simulink model "Quad_F450_Model"  (R2023a)
settings: Solver=FixedStepAuto  StartTime=0.0  StopTime=inf  FixedStep=Copter.SimTs  RelTol=1e-3
InitFcn:
  | load("motor_data.mat")
  | run("Parameters.m")
undefined symbols (not defined in the file or in its folder): Controller, Copter, DiscIntNeverNeededParam, Earth, init, Keyboard, motor_data, w_der_filt, WGS84
libraries: sharedutil x12, slpidlib x8, sharedtransform x5, aerolibpropulsionsys x4, simulink_extras x3, matrix_library x3, shared6dof x1, aerolibtransform2 x1, aerolibatmos2 x1, aerolibsim3d x1, sim3dlib x1
(part 2 of 3)

== system Quad_F450_Model/Copter Properties/Arm_1 ==
  Bus Creator : BusCreator  Inputs=15
  Constant : Constant  Value=Copter.Arm1.Prop.R_m
  Constant1 : Constant  Value=Copter.Arm1.Prop.chord_m
  Constant10 : Constant  Value=Copter.Arm1.defect_rad
  Constant11 : Constant  Value=Copter.Arm1.Prop.Izz_kgm2
  Constant12 : Constant  Value=Copter.Arm1.Motor.time_constant_s
  Constant13 : Constant  Value=Copter.Arm1.Motor.pwm2rpm
  Constant14 : Constant  Value=Copter.Arm1.Prop.Direction
  Constant15 : Constant  Value=Copter.Arm1.h_cg2prop_m
  Constant2 : Constant  Value=Copter.Arm1.Prop.no_of_blades
  Constant3 : Constant  Value=Copter.Arm1.Prop.CT
  Constant4 : Constant  Value=Copter.Arm1.Prop.CQ
  Constant5 : Constant  Value=Copter.Arm1.Prop.flappingOffset_m
  Constant6 : Constant  Value=Copter.Arm1.Prop.Cl_alpha
  Constant7 : Constant  Value=Copter.Arm1.Prop.lock
  Constant8 : Constant  Value=Copter.Arm1.Prop.thetaTip_rad
  Constant9 : Constant  Value=Copter.Arm1.length_m
  Gain : Gain
  Gain1 : Gain
  Matrix Concatenate : Concatenate  NumInputs=3  ConcatenateDimension=2
  Arm_1 : Outport
  wires:
  Constant4/1 -> Bus Creator/10  "prop1_cq"
  Constant8/1 -> Bus Creator/14  "prop1_theta_tip_rad"
  Constant/1 -> Bus Creator/6  "prop1_radius_m"
  Constant2/1 -> Bus Creator/8  "prop1_no_of_blades"
  Constant3/1 -> Bus Creator/9  "prop1_ct"
  Constant6/1 -> Bus Creator/12  "prop1_Cl_alpha"
  Constant1/1 -> Bus Creator/7  "prop1_chord_m"
  Constant5/1 -> Bus Creator/11  "prop1_flapping_offset_m"
  Constant7/1 -> Bus Creator/13  "prop1_lock"
  Constant10/1 -> Bus Creator/2  "arm1_defect_rad"
  Constant11/1 -> Bus Creator/3  "prop1_Izz_kgm2"
  Constant12/1 -> Bus Creator/4  "motor1_time_constant_s"
  Constant13/1 -> Bus Creator/5  "motor1_pwm2rpm"
  Bus Creator/1 -> Arm_1/1
  Constant14/1 -> Bus Creator/15  "prop1_direction"
  Constant9/1 -> Gain1/1, Gain/1  "arm1_length_m"
  Constant15/1 -> Matrix Concatenate/3  "arm1_length_m"
  Gain/1 -> Matrix Concatenate/1
  Gain1/1 -> Matrix Concatenate/2
  Matrix Concatenate/1 -> Bus Creator/1  "cg2motor_arm1_m"

== system Quad_F450_Model/Copter Properties/Arm_2 ==
  Bus Creator : BusCreator  Inputs=15
  Constant : Constant  Value=Copter.Arm2.Prop.R_m
  Constant1 : Constant  Value=Copter.Arm2.Prop.chord_m
  Constant10 : Constant  Value=Copter.Arm2.defect_rad
  Constant11 : Constant  Value=Copter.Arm2.Prop.Izz_kgm2
  Constant12 : Constant  Value=Copter.Arm2.Motor.time_constant_s
  Constant13 : Constant  Value=Copter.Arm2.Motor.pwm2rpm
  Constant14 : Constant  Value=Copter.Arm2.Prop.Direction
  Constant15 : Constant  Value=Copter.Arm2.h_cg2prop_m
  Constant2 : Constant  Value=Copter.Arm2.Prop.no_of_blades
  Constant3 : Constant  Value=Copter.Arm2.Prop.CT
  Constant4 : Constant  Value=Copter.Arm2.Prop.CQ
  Constant5 : Constant  Value=Copter.Arm2.Prop.flappingOffset_m
  Constant6 : Constant  Value=Copter.Arm2.Prop.Cl_alpha
  Constant7 : Constant  Value=Copter.Arm2.Prop.lock
  Constant8 : Constant  Value=Copter.Arm2.Prop.thetaTip_rad
  Constant9 : Constant  Value=Copter.Arm2.length_m
  Gain : Gain  Gain=-1
  Gain1 : Gain  Gain=-1
  Matrix Concatenate : Concatenate  NumInputs=3  ConcatenateDimension=2
  Arm_2 : Outport
  wires:
  Constant4/1 -> Bus Creator/10  "prop2_cq"
  Constant8/1 -> Bus Creator/14  "prop2_theta_tip_rad"
  Constant/1 -> Bus Creator/6  "prop2_radius_m"
  Constant2/1 -> Bus Creator/8  "prop2_no_of_blades"
  Constant3/1 -> Bus Creator/9  "prop2_ct"
  Constant6/1 -> Bus Creator/12  "prop2_Cl_alpha"
  Constant1/1 -> Bus Creator/7  "prop2_chord_m"
  Constant5/1 -> Bus Creator/11  "prop2_flapping_offset_m"
  Constant7/1 -> Bus Creator/13  "prop2_lock"
  Constant10/1 -> Bus Creator/2  "arm2_defect_rad"
  Constant11/1 -> Bus Creator/3  "prop2_Izz_kgm2"
  Constant12/1 -> Bus Creator/4  "motor2_time_constant_s"
  Constant13/1 -> Bus Creator/5  "motor2_pwm2rpm"
  Bus Creator/1 -> Arm_2/1
  Constant14/1 -> Bus Creator/15  "prop2_direction"
  Constant9/1 -> Gain1/1, Gain/1  "arm2_length_m"
  Constant15/1 -> Matrix Concatenate/3  "arm2_length_m"
  Gain/1 -> Matrix Concatenate/1
  Gain1/1 -> Matrix Concatenate/2
  Matrix Concatenate/1 -> Bus Creator/1  "cg2motor_arm2_m"

== system Quad_F450_Model/Copter Properties/Arm_3 ==
  Bus Creator : BusCreator  Inputs=15
  Constant : Constant  Value=Copter.Arm3.Prop.R_m
  Constant1 : Constant  Value=Copter.Arm3.Prop.chord_m
  Constant10 : Constant  Value=Copter.Arm3.defect_rad
  Constant11 : Constant  Value=Copter.Arm3.Prop.Izz_kgm2
  Constant12 : Constant  Value=Copter.Arm3.Motor.time_constant_s
  Constant13 : Constant  Value=Copter.Arm3.Motor.pwm2rpm
  Constant14 : Constant  Value=Copter.Arm3.Prop.Direction
  Constant15 : Constant  Value=Copter.Arm3.h_cg2prop_m
  Constant2 : Constant  Value=Copter.Arm3.Prop.no_of_blades
  Constant3 : Constant  Value=Copter.Arm3.Prop.CT
  Constant4 : Constant  Value=Copter.Arm3.Prop.CQ
  Constant5 : Constant  Value=Copter.Arm3.Prop.flappingOffset_m
  Constant6 : Constant  Value=Copter.Arm3.Prop.Cl_alpha
  Constant7 : Constant  Value=Copter.Arm3.Prop.lock
  Constant8 : Constant  Value=Copter.Arm3.Prop.thetaTip_rad
  Constant9 : Constant  Value=Copter.Arm3.length_m
  Gain : Gain
  Gain1 : Gain  Gain=-1
  Matrix Concatenate : Concatenate  NumInputs=3  ConcatenateDimension=2
  Arm_3 : Outport
  wires:
  Constant4/1 -> Bus Creator/10  "prop3_cq"
  Constant8/1 -> Bus Creator/14  "prop3_theta_tip_rad"
  Constant/1 -> Bus Creator/6  "prop3_radius_m"
  Constant2/1 -> Bus Creator/8  "prop3_no_of_blades"
  Constant3/1 -> Bus Creator/9  "prop3_ct"
  Constant6/1 -> Bus Creator/12  "prop3_Cl_alpha"
  Constant1/1 -> Bus Creator/7  "prop3_chord_m"
  Constant5/1 -> Bus Creator/11  "prop3_flapping_offset_m"
  Constant7/1 -> Bus Creator/13  "prop3_lock"
  Constant10/1 -> Bus Creator/2  "arm3_defect_rad"
  Constant11/1 -> Bus Creator/3  "prop3_Izz_kgm2"
  Constant12/1 -> Bus Creator/4  "motor3_time_constant_s"
  Constant13/1 -> Bus Creator/5  "motor3_pwm2rpm"
  Bus Creator/1 -> Arm_3/1
  Constant14/1 -> Bus Creator/15  "prop3_direction"
  Constant9/1 -> Gain1/1, Gain/1  "arm3_length_m"
  Constant15/1 -> Matrix Concatenate/3  "arm3_length_m"
  Gain/1 -> Matrix Concatenate/1
  Gain1/1 -> Matrix Concatenate/2
  Matrix Concatenate/1 -> Bus Creator/1  "cg2motor_arm3_m"

== system Quad_F450_Model/Copter Properties/Arm_4 ==
  Bus Creator : BusCreator  Inputs=15
  Constant : Constant  Value=Copter.Arm4.Prop.R_m
  Constant1 : Constant  Value=Copter.Arm4.Prop.chord_m
  Constant10 : Constant  Value=Copter.Arm4.defect_rad
  Constant11 : Constant  Value=Copter.Arm4.Prop.Izz_kgm2
  Constant12 : Constant  Value=Copter.Arm4.Motor.time_constant_s
  Constant13 : Constant  Value=Copter.Arm4.Motor.pwm2rpm
  Constant14 : Constant  Value=Copter.Arm4.Prop.Direction
  Constant15 : Constant  Value=Copter.Arm4.h_cg2prop_m
  Constant2 : Constant  Value=Copter.Arm4.Prop.no_of_blades
  Constant3 : Constant  Value=Copter.Arm4.Prop.CT
  Constant4 : Constant  Value=Copter.Arm4.Prop.CQ
  Constant5 : Constant  Value=Copter.Arm4.Prop.flappingOffset_m
  Constant6 : Constant  Value=Copter.Arm4.Prop.Cl_alpha
  Constant7 : Constant  Value=Copter.Arm4.Prop.lock
  Constant8 : Constant  Value=Copter.Arm4.Prop.thetaTip_rad
  Constant9 : Constant  Value=Copter.Arm4.length_m
  Gain : Gain  Gain=-1
  Gain1 : Gain
  Matrix Concatenate : Concatenate  NumInputs=3  ConcatenateDimension=2
  Arm_4 : Outport
  wires:
  Constant4/1 -> Bus Creator/10  "prop4_cq"
  Constant8/1 -> Bus Creator/14  "prop4_theta_tip_rad"
  Constant/1 -> Bus Creator/6  "prop4_radius_m"
  Constant2/1 -> Bus Creator/8  "prop4_no_of_blades"
  Constant3/1 -> Bus Creator/9  "prop4_ct"
  Constant6/1 -> Bus Creator/12  "prop4_Cl_alpha"
  Constant1/1 -> Bus Creator/7  "prop4_chord_m"
  Constant5/1 -> Bus Creator/11  "prop4_flapping_offset_m"
  Constant7/1 -> Bus Creator/13  "prop4_lock"
  Constant10/1 -> Bus Creator/2  "arm4_defect_rad"
  Constant11/1 -> Bus Creator/3  "prop4_Izz_kgm2"
  Constant12/1 -> Bus Creator/4  "motor4_time_constant_s"
  Constant13/1 -> Bus Creator/5  "motor4_pwm2rpm"
  Bus Creator/1 -> Arm_4/1
  Constant14/1 -> Bus Creator/15  "prop4_direction"
  Constant9/1 -> Gain1/1, Gain/1  "arm4_length_m"
  Constant15/1 -> Matrix Concatenate/3  "arm4_length_m"
  Gain/1 -> Matrix Concatenate/1
  Gain1/1 -> Matrix Concatenate/2
  Matrix Concatenate/1 -> Bus Creator/1  "cg2motor_arm4_m"

== system Quad_F450_Model/Copter Properties/Subsystem ==
  Bus Creator : BusCreator  Inputs=7
  Constant1 : Constant  Value=Copter.inertia_matrix_kgm2
  Constant2 : Constant  Value=Copter.S_area_m2
  Constant3 : Constant  Value=Copter.Cd
  Constant4 : Constant  Value=Copter.Ryz_cg2ac_m
  Constant5 : Constant  Value=Copter.Rxz_cg2ac_m
  Constant6 : Constant  Value=Copter.Rxy_cg2ac_m
  Constant9 : Constant  Value=Copter.mass_kg
  Copter_Frame : Outport
  wires:
  Constant9/1 -> Bus Creator/1  "mass_kg"
  Constant1/1 -> Bus Creator/2  "inertia_matrix_kgm2"
  Constant2/1 -> Bus Creator/3  "S_area_m2"
  Constant3/1 -> Bus Creator/4  "Cd"
  Constant4/1 -> Bus Creator/5  "Ryz_cg2ac_m"
  Bus Creator/1 -> Copter_Frame/1
  Constant5/1 -> Bus Creator/6  "Rxz_cg2ac_m"
  Constant6/1 -> Bus Creator/7  "Rxy_cg2ac_m"

== system Quad_F450_Model/DYNAMIC_MODEL/Aerodynamic Forces and Moments ==
  V_air_ms : Inport
  Environment : Inport  Port=2
  Copter : Inport  Port=3
  Add : Sum  Inputs=3
  Bus Selector : BusSelector  OutputSignals=Frame.S_area_m2,Frame.Cd,Frame.Rxy_cg2ac_m,Frame.Rxz_cg2ac_m,Frame.Ryz_cg2ac_m
  Bus Selector1 : BusSelector  OutputSignals=Atmosphere_Prop.air_density_kgm3
  Constant : Constant  Value=0
  Constant1 : Constant  Value=0
  Constant2 : Constant  Value=0
  Cross Product : matrix_library/Cross Product
  Cross Product1 : matrix_library/Cross Product
  Cross Product2 : matrix_library/Cross Product
  Gain : Gain  Gain=-1
  Gain1 : Gain  Gain=1/2
  Mux : Mux  Inputs=3
  Mux1 : Mux  Inputs=3
  Mux2 : Mux  Inputs=3
  Product : Product  Inputs=5
  Selector : Selector  InputPortWidth=3  IndexOptions=Index vector (dialog)  Indices=1  OutputSizes=1
  Selector1 : Selector  InputPortWidth=3  IndexOptions=Index vector (dialog)  Indices=2  OutputSizes=1
  Selector2 : Selector  InputPortWidth=3  IndexOptions=Index vector (dialog)  Indices=3  OutputSizes=1
  Sign : Signum
  Square : Math  Operator=square
  F_aero_b_N : Outport
  M_aero_b_Nm : Outport  Port=2
  wires:
  Square/1 -> Gain1/1
  V_air_ms/1 -> Square/1, Sign/1
  [S_m2] -> Product/4
  [Cd] -> Product/5
  [rho_kgm3] -> Product/3
  Gain1/1 -> Product/2
  Copter/1 -> Bus Selector/1
  Bus Selector/3 -> [Rxy_cg2ac_m]  "<Rxy_cg2ac_m>"
  Bus Selector/2 -> [Cd]  "<Cd>"
  Bus Selector/1 -> [S_m2]  "<S_area_m2>"
  Environment/1 -> Bus Selector1/1
  Bus Selector1/1 -> [rho_kgm3]  "<air_density_kgm3>"
  Bus Selector/4 -> [Rxz_cg2ac_m]  "<Rxz_cg2ac_m>"
  Bus Selector/5 -> [Ryz_cg2ac_m]  "<Ryz_cg2ac_m>"
  Product/1 -> Gain/1
  [F_aero_b_N] -> F_aero_b_N/1
  [F_aero_b_N] -> Selector/1
  Selector/1 -> Mux/1
  Constant/1 -> Mux/3, Mux/2
  Mux/1 -> Cross Product/2
  [Ryz_cg2ac_m] -> Cross Product/1
  [Rxz_cg2ac_m] -> Cross Product1/1
  Mux1/1 -> Cross Product1/2
  [F_aero_b_N] -> Selector1/1
  [F_aero_b_N] -> Selector2/1
  Mux2/1 -> Cross Product2/2
  [Rxy_cg2ac_m] -> Cross Product2/1
  Selector2/1 -> Mux2/3
  Constant2/1 -> Mux2/1, Mux2/2
  Selector1/1 -> Mux1/2
  Constant1/1 -> Mux1/3, Mux1/1
  Cross Product1/1 -> Add/2
  Cross Product2/1 -> Add/3
  Cross Product/1 -> Add/1
  Add/1 -> M_aero_b_Nm/1
  Sign/1 -> Product/1
  Gain/1 -> [F_aero_b_N]

== system Quad_F450_Model/DYNAMIC_MODEL/Gravity Force  ==
  dcm_e2b : Inport
  Environment : Inport  Port=2
  Copter : Inport  Port=3
  Bus Selector : BusSelector  OutputSignals=Frame.mass_kg
  Bus Selector1 : BusSelector  OutputSignals=gravity_e_mss
  Matrix Multiply : Product  Multiplication=Matrix(*)
  Product : Product
  F_grav_b_N : Outport
  wires:
  dcm_e2b/1 -> Matrix Multiply/1
  Environment/1 -> Bus Selector1/1
  Matrix Multiply/1 -> Product/1
  Product/1 -> F_grav_b_N/1
  Copter/1 -> Bus Selector/1
  Bus Selector/1 -> Product/2  "<mass_kg>"
  Bus Selector1/1 -> Matrix Multiply/2  "<gravity_e_mss>"

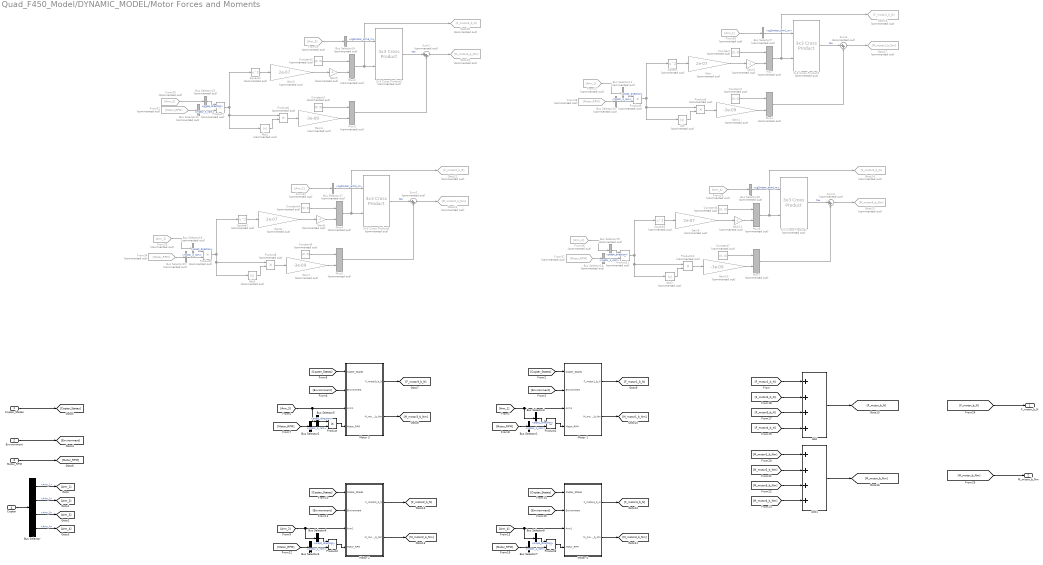
== system Quad_F450_Model/DYNAMIC_MODEL/Motor Forces and Moments ==
  Copter_States : Inport
  Environment : Inport  Port=2
  Motor_RPM : Inport  Port=3
  Copter : Inport  Port=4
  3x3 Cross Product{1..4} (4 alike) : sharedutil/3x3 Cross Product  Commented=on  aMode=aMode
      settings: LibrarySourceBlock=aerolibpropulsionsys/Rotor Subsystem/3x3 Cross Product1
  Abs{,1..3} (4 alike) : Abs  Commented=on  SaturateOnIntegerOverflow=off
  Add : Sum  Inputs=4
  Add1 : Sum  Inputs=4
  Bus Selector : BusSelector  OutputSignals=Arm_1,Arm_2,Arm_3,Arm_4
  Bus Selector1 : BusSelector  OutputSignals=motor_1_rpm
  Bus Selector10 : BusSelector  Commented=on  OutputSignals=motor_1_rpm
  Bus Selector11 : BusSelector  Commented=on  OutputSignals=prop1_direction
  Bus Selector12 : BusSelector  Commented=on  OutputSignals=motor_3_rpm
  Bus Selector13 : BusSelector  Commented=on  OutputSignals=prop3_direction
  Bus Selector14 : BusSelector  Commented=on  OutputSignals=cg2motor_arm3_m
  Bus Selector15 : BusSelector  Commented=on  OutputSignals=motor_2_rpm
  Bus Selector16 : BusSelector  Commented=on  OutputSignals=prop2_direction
  Bus Selector17 : BusSelector  Commented=on  OutputSignals=cg2motor_arm2_m
  Bus Selector18 : BusSelector  Commented=on  OutputSignals=motor_4_rpm
  Bus Selector19 : BusSelector  Commented=on  OutputSignals=prop4_direction
  Bus Selector2 : BusSelector  OutputSignals=motor_3_rpm
  Bus Selector20 : BusSelector  Commented=on  OutputSignals=cg2motor_arm4_m
  Bus Selector3 : BusSelector  OutputSignals=prop1_direction
  Bus Selector4 : BusSelector  OutputSignals=motor_2_rpm
  Bus Selector5 : BusSelector  OutputSignals=prop3_direction
  Bus Selector6 : BusSelector  OutputSignals=prop2_direction
  Bus Selector7 : BusSelector  OutputSignals=motor_4_rpm
  Bus Selector8 : BusSelector  OutputSignals=prop4_direction
  Bus Selector9 : BusSelector  Commented=on  OutputSignals=cg2motor_arm1_m
  Constant{,1..7} (8 alike) : Constant  Commented=on  Value=[0; 0]
  From26 : From  Commented=on  GotoTag=Arm_1
  From27 : From  Commented=on  GotoTag=Arm_1
  From{28,31,34,37} (4 alike) : From  Commented=on  GotoTag=Motor_RPM
  From29 : From  Commented=on  GotoTag=Arm_3
  From30 : From  Commented=on  GotoTag=Arm_3
  From32 : From  Commented=on  GotoTag=Arm_2
  From33 : From  Commented=on  GotoTag=Arm_2
  From35 : From  Commented=on  GotoTag=Arm_4
  From36 : From  Commented=on  GotoTag=Arm_4
  Gain{,3,6,9} (4 alike) : Gain  Commented=on  Gain=2e-07
  Gain{1,4,7,10} (4 alike) : Gain  Commented=on  Gain=-3e-09
  Gain{2,5,8,11} (4 alike) : Gain  Commented=on  Gain=-1
  Goto17 : Goto  Commented=on  GotoTag=M_motor1_b_Nm
  Goto18 : Goto  Commented=on  GotoTag=F_motor1_b_N
  Goto19 : Goto  Commented=on  GotoTag=M_motor3_b_Nm
  Goto20 : Goto  Commented=on  GotoTag=F_motor3_b_N
  Goto21 : Goto  Commented=on  GotoTag=M_motor2_b_Nm
  Goto22 : Goto  Commented=on  GotoTag=F_motor2_b_N
  Goto23 : Goto  Commented=on  GotoTag=M_motor4_b_Nm
  Goto24 : Goto  Commented=on  GotoTag=F_motor4_b_N
  Motor 1 : Subsystem
  Motor 2 : Subsystem
  Motor 3 : Subsystem
  Motor 4 : Subsystem
  Mux{,1..7} (8 alike) : Mux  Commented=on  Inputs=2
  Product{,1..3} (4 alike) : Product
  Product{4..11} (8 alike) : Product  Commented=on
  Square{,1..3} (4 alike) : Math  Commented=on  Operator=square
  Sum{1..4} (4 alike) : Sum  Commented=on  Inputs=|++  OutDataTypeStr=Inherit: Inherit via back propagation
  F_motor_b_N : Outport
  M_motor_b_Nm : Outport  Port=2
  wires:
  Copter/1 -> Bus Selector/1
  Bus Selector/1 -> [Arm_1]  "<Arm_1>"
  Bus Selector/2 -> [Arm_2]  "<Arm_2>"
  Bus Selector/3 -> [Arm_3]  "<Arm_3>"
  Bus Selector/4 -> [Arm_4]  "<Arm_4>"
  Environment/1 -> [Environment]
  Copter_States/1 -> [Copter_States]
  Motor_RPM/1 -> [Motor_RPM]
  [Copter_States] -> Motor 3/1(Copter_States)
  [Motor_RPM] -> Bus Selector2/1
  [Environment] -> Motor 3/2(Environment)
  Bus Selector2/1 -> Product/2  "<motor_3_rpm>"
  Product/1 -> Motor 3/4(Motor_RPM)
  [Arm_3] -> Bus Selector5/1, Motor 3/3(Arm1)
  Bus Selector5/1 -> Product/1  "<prop3_direction>"
  Bus Selector1/1 -> Product1/2  "<motor_1_rpm>"
  Product1/1 -> Motor 1/4(Motor_RPM)
  [Arm_1] -> Bus Selector3/1, Motor 1/3(Arm1)
  [Motor_RPM] -> Bus Selector1/1
  [Copter_States] -> Motor 1/1(Copter_States)
  [Environment] -> Motor 1/2(Environment)
  Bus Selector3/1 -> Product1/1  "<prop1_direction>"
  Bus Selector4/1 -> Product2/2  "<motor_2_rpm>"
  Product2/1 -> Motor 2/4(Motor_RPM)
  [Arm_2] -> Bus Selector6/1, Motor 2/3(Arm1)
  [Motor_RPM] -> Bus Selector4/1
  [Copter_States] -> Motor 2/1(Copter_States)
  [Environment] -> Motor 2/2(Environment)
  Bus Selector6/1 -> Product2/1  "<prop2_direction>"
  Bus Selector7/1 -> Product3/2  "<motor_4_rpm>"
  Product3/1 -> Motor 4/4(Motor_RPM)
  [Arm_4] -> Bus Selector8/1, Motor 4/3(Arm1)
  [Motor_RPM] -> Bus Selector7/1
  [Copter_States] -> Motor 4/1(Copter_States)
  [Environment] -> Motor 4/2(Environment)
  Bus Selector8/1 -> Product3/1  "<prop4_direction>"
  Motor 3/1(F_motor3_b_N) -> [F_motor3_b_N]
  Motor 3/2(M_motor3_b_Nm) -> [M_motor3_b_Nm]
  Motor 1/1(F_motor1_b_N) -> [F_motor1_b_N]
  Motor 1/2(M_motor1_b_Nm) -> [M_motor1_b_Nm]
  Motor 4/1(F_motor4_b_N) -> [F_motor4_b_N]
  Motor 4/2(M_motor4_b_Nm) -> [M_motor4_b_Nm]
  Motor 2/1(F_motor2_b_N) -> [F_motor2_b_N]
  Motor 2/2(M_motor2_b_Nm) -> [M_motor2_b_Nm]
  [F_motor1_b_N] -> Add/1
  [F_motor2_b_N] -> Add/2
  [F_motor3_b_N] -> Add/3
  [F_motor4_b_N] -> Add/4
  [M_motor1_b_Nm] -> Add1/1
  [M_motor2_b_Nm] -> Add1/2
  [M_motor3_b_Nm] -> Add1/3
  [M_motor4_b_Nm] -> Add1/4
  Add/1 -> [F_motor_b_N]
  Add1/1 -> [M_motor_b_Nm]
  [F_motor_b_N] -> F_motor_b_N/1
  [M_motor_b_Nm] -> M_motor_b_Nm/1
  3x3 Cross Product1/1 -> Sum4/1  "tau"
  Square/1 -> Gain/1
  Gain/1 -> Gain2/1
  Constant/1 -> Mux/1
  Mux/1 -> Goto18/1, 3x3 Cross Product1/2
  From26/1 -> Bus Selector9/1
  Bus Selector9/1 -> 3x3 Cross Product1/1  "<cg2motor_arm1_m>"
  Constant1/1 -> Mux1/1
  Gain1/1 -> Mux1/2
  Product4/1 -> Gain1/1
  Abs/1 -> Product4/2
  Mux1/1 -> Sum4/2
  Gain2/1 -> Mux/2
  Sum4/1 -> Goto17/1
  From27/1 -> Bus Selector11/1
  From28/1 -> Bus Selector10/1
  Bus Selector10/1 -> Product5/2  "<motor_1_rpm>"
  Bus Selector11/1 -> Product5/1  "<prop1_direction>"
  Product5/1 -> Square/1, Abs/1, Product4/1
  Product7/1 -> Product6/1, Abs1/1, Square1/1
  Bus Selector13/1 -> Product7/1  "<prop3_direction>"
  Bus Selector12/1 -> Product7/2  "<motor_3_rpm>"
  From31/1 -> Bus Selector12/1
  From30/1 -> Bus Selector13/1
  Sum1/1 -> Goto19/1
  Gain5/1 -> Mux2/2
  Mux3/1 -> Sum1/2
  Abs1/1 -> Product6/2
  Product6/1 -> Gain4/1
  Gain4/1 -> Mux3/2
  Constant3/1 -> Mux3/1
  Bus Selector14/1 -> 3x3 Cross Product2/1  "<cg2motor_arm3_m>"
  From29/1 -> Bus Selector14/1
  Mux2/1 -> 3x3 Cross Product2/2, Goto20/1
  Constant2/1 -> Mux2/1
  Gain3/1 -> Gain5/1
  Square1/1 -> Gain3/1
  3x3 Cross Product2/1 -> Sum1/1  "tau"
  3x3 Cross Product3/1 -> Sum2/1  "tau"
  Square2/1 -> Gain6/1
  Gain6/1 -> Gain8/1
  Constant4/1 -> Mux4/1
  Mux4/1 -> Goto22/1, 3x3 Cross Product3/2
  From32/1 -> Bus Selector17/1
  Bus Selector17/1 -> 3x3 Cross Product3/1  "<cg2motor_arm2_m>"
  Constant5/1 -> Mux5/1
  Gain7/1 -> Mux5/2
  Product8/1 -> Gain7/1
  Abs2/1 -> Product8/2
  Mux5/1 -> Sum2/2
  Gain8/1 -> Mux4/2
  Sum2/1 -> Goto21/1
  From33/1 -> Bus Selector16/1
  From34/1 -> Bus Selector15/1
  Bus Selector15/1 -> Product9/2  "<motor_2_rpm>"
  Bus Selector16/1 -> Product9/1  "<prop2_direction>"
  Product9/1 -> Square2/1, Abs2/1, Product8/1
  Product11/1 -> Product10/1, Abs3/1, Square3/1
  Bus Selector19/1 -> Product11/1  "<prop4_direction>"
  Bus Selector18/1 -> Product11/2  "<motor_4_rpm>"
  From37/1 -> Bus Selector18/1
  From36/1 -> Bus Selector19/1
  Sum3/1 -> Goto23/1
  Gain11/1 -> Mux6/2
  Mux7/1 -> Sum3/2
  Abs3/1 -> Product10/2
  Product10/1 -> Gain10/1
  Gain10/1 -> Mux7/2
  Constant7/1 -> Mux7/1
  Bus Selector20/1 -> 3x3 Cross Product4/1  "<cg2motor_arm4_m>"
  From35/1 -> Bus Selector20/1
  Mux6/1 -> 3x3 Cross Product4/2, Goto24/1
  Constant6/1 -> Mux6/1
  Gain9/1 -> Gain11/1
  Square3/1 -> Gain9/1
  3x3 Cross Product4/1 -> Sum3/1  "tau"

== system Quad_F450_Model/DYNAMIC_MODEL/Motor_1 ==
  in : Inport
  tau : Inport  Port=2
  reset : Inport  Port=3
  Integrator : Integrator  ExternalReset=rising  InitialCondition=init.rpm(1)
  Product : Product
  Reciprocal : Product  Inputs=/
  Sum : Sum  Inputs=|+-
  out : Outport
  wires:
  Integrator/1 -> out/1, Sum/2
  Sum/1 -> Product/2
  tau/1 -> Reciprocal/1
  Product/1 -> Integrator/1
  Reciprocal/1 -> Product/1
  reset/1 -> Integrator/2
  in/1 -> Sum/1

== system Quad_F450_Model/DYNAMIC_MODEL/Motor_2 ==
  in : Inport
  tau : Inport  Port=2
  reset : Inport  Port=3
  Integrator : Integrator  ExternalReset=rising  InitialCondition=init.rpm(2)
  Product : Product
  Reciprocal : Product  Inputs=/
  Sum : Sum  Inputs=|+-
  out : Outport
  wires:
  Integrator/1 -> out/1, Sum/2
  Sum/1 -> Product/2
  tau/1 -> Reciprocal/1
  Product/1 -> Integrator/1
  Reciprocal/1 -> Product/1
  reset/1 -> Integrator/2
  in/1 -> Sum/1

== system Quad_F450_Model/DYNAMIC_MODEL/Motor_3 ==
  in : Inport
  tau : Inport  Port=2
  reset : Inport  Port=3
  Integrator : Integrator  ExternalReset=rising  InitialCondition=init.rpm(3)
  Product : Product
  Reciprocal : Product  Inputs=/
  Sum : Sum  Inputs=|+-
  out : Outport
  wires:
  in/1 -> Sum/1
  reset/1 -> Integrator/2
  Reciprocal/1 -> Product/1
  Product/1 -> Integrator/1
  tau/1 -> Reciprocal/1
  Sum/1 -> Product/2
  Integrator/1 -> Sum/2, out/1

== system Quad_F450_Model/DYNAMIC_MODEL/Motor_4 ==
  in : Inport
  tau : Inport  Port=2
  reset : Inport  Port=3
  Integrator : Integrator  ExternalReset=rising  InitialCondition=init.rpm(4)
  Product : Product
  Reciprocal : Product  Inputs=/
  Sum : Sum  Inputs=|+-
  out : Outport
  wires:
  in/1 -> Sum/1
  reset/1 -> Integrator/2
  Reciprocal/1 -> Product/1
  Product/1 -> Integrator/1
  tau/1 -> Reciprocal/1
  Sum/1 -> Product/2
  Integrator/1 -> Sum/2, out/1

== system Quad_F450_Model/ENVIRONMENT/Subsystem ==
  Constant : Constant  Value=zeros(3,1)
  wind_vel_ms : Outport
  wires:
  Constant/1 -> wind_vel_ms/1

== system Quad_F450_Model/DYNAMIC_MODEL/Motor Forces and Moments/Motor 1 ==
  Copter_States : Inport
  Environment : Inport  Port=2
  Arm1 : Inport  Port=3
  Motor_RPM : Inport  Port=4
  3x3 Cross Product1 : sharedutil/3x3 Cross Product  aMode=aMode
      settings: LibrarySourceBlock=aerolibpropulsionsys/Rotor Subsystem/3x3 Cross Product1
  Bus Selector : BusSelector  OutputSignals=vel_b_ms,angular_vel_b_rads
  Bus Selector1 : BusSelector  OutputSignals=cg2motor_arm1_m,prop1_Izz_kgm2
  Bus Selector2 : BusSelector  OutputSignals=Atmosphere_Prop.air_density_kgm3
  Derivative : Derivative  CoefficientInTFapproximation=1/10
  Forces : Subsystem
  Gain : Gain  Gain=2*pi/60
  Gain1 : Gain  Gain=-1
  Gain2 : Gain  Gain=Copter.Gyroscopic_Effect_Active
  Moments : Subsystem
  Mux : Mux  Inputs=3
  Product : Product
  Product1 : Product
  Product2 : Product
  Selector : Selector  InputPortWidth=3  IndexOptions=Index vector (dialog)  Indices=1  OutputSizes=1
  Selector1 : Selector  InputPortWidth=3  IndexOptions=Index vector (dialog)  Indices=2  OutputSizes=1
  Subsystem : Subsystem
  Sum4 : Sum  Inputs=+++  OutDataTypeStr=Inherit: Inherit via back propagation
  Transfer Fcn : TransferFcn  Numerator=[w_der_filt]  Denominator=[1 w_der_filt]
  F_motor1_b_N : Outport  OutDataTypeStr=double  VectorParamsAs1DForOutWhenUnconnected=off
  M_motor1_b_Nm : Outport  Port=2  OutDataTypeStr=double  VectorParamsAs1DForOutWhenUnconnected=off
  wires:
  Sum4/1 -> M_motor1_b_Nm/1
  Forces/1(Fxyz) -> F_motor1_b_N/1, 3x3 Cross Product1/2
  Subsystem/1(a1s) -> Forces/1(a1s)
  Subsystem/2(b1s) -> Forces/2(b1s)
  Copter_States/1 -> Bus Selector/1
  Arm1/1 -> [Arm], Bus Selector1/1
  Bus Selector1/1 -> [ArmL]  "<cg2motor_arm1_m>"
  [ArmL] -> 3x3 Cross Product1/1
  Environment/1 -> Bus Selector2/1
  Bus Selector2/1 -> [rho]  "<air_density_kgm3>"
  [rho] -> Forces/4(rho)
  [Arm] -> Subsystem/4(Arm)
  [Arm] -> Forces/5(Arm)
  [rho] -> Moments/1(rho)
  [Arm] -> Moments/3(Arm)
  Motor_RPM/1 -> Gain/1
  Gain/1 -> [w_rads]
  [w_rads] -> Subsystem/3(w)
  [w_rads] -> Moments/2(w)
  [w_rads] -> Forces/3(w)
  Bus Selector/1 -> [Vb_ms]  "<vel_b_ms>"
  Bus Selector/2 -> [pqr_rads]  "<angular_vel_b_rads>"
  [pqr_rads] -> Subsystem/2(pqr)
  [Vb_ms] -> Subsystem/1(Vb)
  Gain1/1 -> Mux/2
  Product/1 -> Gain1/1
  [w_rads] -> Derivative/1, Product1/2, Product/1
  [pqr_rads] -> Selector1/1, Selector/1
  Selector/1 -> Product/2
  Product1/1 -> Mux/1
  Selector1/1 -> Product1/1
  Derivative/1 -> Transfer Fcn/1
  Mux/1 -> Product2/1
  [Iz_prop_kgm2] -> Product2/2
  3x3 Cross Product1/1 -> Sum4/2  "tau"
  Moments/1(Mxyz) -> Sum4/3
  Product2/1 -> Gain2/1
  Bus Selector1/2 -> [Iz_prop_kgm2]  "<prop1_Izz_kgm2>"
  Transfer Fcn/1 -> Mux/3
  Gain2/1 -> Sum4/1

== system Quad_F450_Model/DYNAMIC_MODEL/Motor Forces and Moments/Motor 2 ==
  Copter_States : Inport
  Environment : Inport  Port=2
  Arm1 : Inport  Port=3
  Motor_RPM : Inport  Port=4
  3x3 Cross Product1 : sharedutil/3x3 Cross Product  aMode=aMode
      settings: LibrarySourceBlock=aerolibpropulsionsys/Rotor Subsystem/3x3 Cross Product1
  Bus Selector : BusSelector  OutputSignals=vel_b_ms,angular_vel_b_rads
  Bus Selector1 : BusSelector  OutputSignals=cg2motor_arm2_m,prop2_Izz_kgm2
  Bus Selector2 : BusSelector  OutputSignals=Atmosphere_Prop.air_density_kgm3
  Derivative : Derivative
  Forces : Subsystem
  Gain : Gain  Gain=2*pi/60
  Gain1 : Gain  Gain=-1
  Gain2 : Gain  Gain=Copter.Gyroscopic_Effect_Active
  Moments : Subsystem
  Mux : Mux  Inputs=3
  Product : Product
  Product1 : Product
  Product2 : Product
  Selector : Selector  InputPortWidth=3  IndexOptions=Index vector (dialog)  Indices=1  OutputSizes=1
  Selector1 : Selector  InputPortWidth=3  IndexOptions=Index vector (dialog)  Indices=2  OutputSizes=1
  Subsystem : Subsystem
  Sum4 : Sum  Inputs=+++  OutDataTypeStr=Inherit: Inherit via back propagation
  Transfer Fcn : TransferFcn  Numerator=[w_der_filt]  Denominator=[1 w_der_filt]
  F_motor2_b_N : Outport  OutDataTypeStr=double  VectorParamsAs1DForOutWhenUnconnected=off
  M_motor2_b_Nm : Outport  Port=2  OutDataTypeStr=double  VectorParamsAs1DForOutWhenUnconnected=off
  wires:
  Sum4/1 -> M_motor2_b_Nm/1
  Forces/1(Fxyz) -> F_motor2_b_N/1, 3x3 Cross Product1/2
  Subsystem/1(a1s) -> Forces/1(a1s)
  Subsystem/2(b1s) -> Forces/2(b1s)
  Copter_States/1 -> Bus Selector/1
  Arm1/1 -> [Arm], Bus Selector1/1
  Bus Selector1/1 -> [ArmL]  "<cg2motor_arm2_m>"
  [ArmL] -> 3x3 Cross Product1/1
  Environment/1 -> Bus Selector2/1
  Bus Selector2/1 -> [rho]  "<air_density_kgm3>"
  [rho] -> Forces/4(rho)
  [Arm] -> Subsystem/4(Arm)
  [Arm] -> Forces/5(Arm)
  [rho] -> Moments/1(rho)
  [Arm] -> Moments/3(Arm)
  Motor_RPM/1 -> Gain/1
  Gain/1 -> [w_rads]
  [w_rads] -> Subsystem/3(w)
  [w_rads] -> Moments/2(w)
  [w_rads] -> Forces/3(w)
  Bus Selector/1 -> [Vb_ms]  "<vel_b_ms>"
  Bus Selector/2 -> [pqr_rads]  "<angular_vel_b_rads>"
  [pqr_rads] -> Subsystem/2(pqr)
  [Vb_ms] -> Subsystem/1(Vb)
  [Iz_prop_kgm2] -> Product2/2
  Product/1 -> Gain1/1
  [w_rads] -> Derivative/1, Product1/2, Product/1
  Product2/1 -> Gain2/1
  Product1/1 -> Mux/1
  Selector/1 -> Product/2
  Mux/1 -> Product2/1
  [pqr_rads] -> Selector1/1, Selector/1
  Gain1/1 -> Mux/2
  Selector1/1 -> Product1/1
  Derivative/1 -> Transfer Fcn/1
  3x3 Cross Product1/1 -> Sum4/2  "tau"
  Moments/1(Mxyz) -> Sum4/3
  Bus Selector1/2 -> [Iz_prop_kgm2]  "<prop2_Izz_kgm2>"
  Transfer Fcn/1 -> Mux/3
  Gain2/1 -> Sum4/1

== system Quad_F450_Model/DYNAMIC_MODEL/Motor Forces and Moments/Motor 3 ==
  Copter_States : Inport
  Environment : Inport  Port=2
  Arm1 : Inport  Port=3
  Motor_RPM : Inport  Port=4
  3x3 Cross Product1 : sharedutil/3x3 Cross Product  aMode=aMode
      settings: LibrarySourceBlock=aerolibpropulsionsys/Rotor Subsystem/3x3 Cross Product1
  Bus Selector : BusSelector  OutputSignals=vel_b_ms,angular_vel_b_rads
  Bus Selector1 : BusSelector  OutputSignals=cg2motor_arm3_m,prop3_Izz_kgm2
  Bus Selector2 : BusSelector  OutputSignals=Atmosphere_Prop.air_density_kgm3
  Derivative : Derivative
  Forces : Subsystem
  Gain : Gain  Gain=2*pi/60
  Gain1 : Gain  Gain=-1
  Gain2 : Gain  Gain=Copter.Gyroscopic_Effect_Active
  Moments : Subsystem
  Mux : Mux  Inputs=3
  Product : Product
  Product1 : Product
  Product2 : Product
  Selector : Selector  InputPortWidth=3  IndexOptions=Index vector (dialog)  Indices=1  OutputSizes=1
  Selector1 : Selector  InputPortWidth=3  IndexOptions=Index vector (dialog)  Indices=2  OutputSizes=1
  Subsystem : Subsystem
  Sum4 : Sum  Inputs=+++  OutDataTypeStr=Inherit: Inherit via back propagation
  Transfer Fcn : TransferFcn  Numerator=[w_der_filt]  Denominator=[1 w_der_filt]
  F_motor3_b_N : Outport  OutDataTypeStr=double  VectorParamsAs1DForOutWhenUnconnected=off
  M_motor3_b_Nm : Outport  Port=2  OutDataTypeStr=double  VectorParamsAs1DForOutWhenUnconnected=off
  wires:
  Sum4/1 -> M_motor3_b_Nm/1
  Forces/1(Fxyz) -> F_motor3_b_N/1, 3x3 Cross Product1/2
  Subsystem/1(a1s) -> Forces/1(a1s)
  Subsystem/2(b1s) -> Forces/2(b1s)
  Copter_States/1 -> Bus Selector/1
  Arm1/1 -> [Arm], Bus Selector1/1
  Bus Selector1/1 -> [ArmL]  "<cg2motor_arm3_m>"
  [ArmL] -> 3x3 Cross Product1/1
  Environment/1 -> Bus Selector2/1
  Bus Selector2/1 -> [rho]  "<air_density_kgm3>"
  [rho] -> Forces/4(rho)
  [Arm] -> Subsystem/4(Arm)
  [Arm] -> Forces/5(Arm)
  [rho] -> Moments/1(rho)
  [Arm] -> Moments/3(Arm)
  Motor_RPM/1 -> Gain/1
  Gain/1 -> [w_rads]
  [w_rads] -> Subsystem/3(w)
  [w_rads] -> Moments/2(w)
  [w_rads] -> Forces/3(w)
  Bus Selector/1 -> [Vb_ms]  "<vel_b_ms>"
  Bus Selector/2 -> [pqr_rads]  "<angular_vel_b_rads>"
  [pqr_rads] -> Subsystem/2(pqr)
  [Vb_ms] -> Subsystem/1(Vb)
  [Iz_prop_kgm2] -> Product2/2
  Product/1 -> Gain1/1
  [w_rads] -> Derivative/1, Product1/2, Product/1
  Product2/1 -> Gain2/1
  Product1/1 -> Mux/1
  Selector/1 -> Product/2
  Mux/1 -> Product2/1
  [pqr_rads] -> Selector1/1, Selector/1
  Gain1/1 -> Mux/2
  Selector1/1 -> Product1/1
  Derivative/1 -> Transfer Fcn/1
  3x3 Cross Product1/1 -> Sum4/2  "tau"
  Moments/1(Mxyz) -> Sum4/3
  Bus Selector1/2 -> [Iz_prop_kgm2]  "<prop3_Izz_kgm2>"
  Transfer Fcn/1 -> Mux/3
  Gain2/1 -> Sum4/1

== system Quad_F450_Model/DYNAMIC_MODEL/Motor Forces and Moments/Motor 4 ==
  Copter_States : Inport
  Environment : Inport  Port=2
  Arm1 : Inport  Port=3
  Motor_RPM : Inport  Port=4
  3x3 Cross Product1 : sharedutil/3x3 Cross Product  aMode=aMode
      settings: LibrarySourceBlock=aerolibpropulsionsys/Rotor Subsystem/3x3 Cross Product1
  Bus Selector : BusSelector  OutputSignals=vel_b_ms,angular_vel_b_rads
  Bus Selector1 : BusSelector  OutputSignals=cg2motor_arm4_m,prop4_Izz_kgm2
  Bus Selector2 : BusSelector  OutputSignals=Atmosphere_Prop.air_density_kgm3
  Derivative : Derivative
  Forces : Subsystem
  Gain : Gain  Gain=2*pi/60
  Gain1 : Gain  Gain=-1
  Gain2 : Gain  Gain=Copter.Gyroscopic_Effect_Active
  Moments : Subsystem
  Mux : Mux  Inputs=3
  Product : Product
  Product1 : Product
  Product2 : Product
  Selector : Selector  InputPortWidth=3  IndexOptions=Index vector (dialog)  Indices=1  OutputSizes=1
  Selector1 : Selector  InputPortWidth=3  IndexOptions=Index vector (dialog)  Indices=2  OutputSizes=1
  Subsystem : Subsystem
  Sum4 : Sum  Inputs=+++  OutDataTypeStr=Inherit: Inherit via back propagation
  Transfer Fcn : TransferFcn  Numerator=[w_der_filt]  Denominator=[1 w_der_filt]
  F_motor4_b_N : Outport  OutDataTypeStr=double  VectorParamsAs1DForOutWhenUnconnected=off
  M_motor4_b_Nm : Outport  Port=2  OutDataTypeStr=double  VectorParamsAs1DForOutWhenUnconnected=off
  wires:
  Sum4/1 -> M_motor4_b_Nm/1
  Forces/1(Fxyz) -> F_motor4_b_N/1, 3x3 Cross Product1/2
  Subsystem/1(a1s) -> Forces/1(a1s)
  Subsystem/2(b1s) -> Forces/2(b1s)
  Copter_States/1 -> Bus Selector/1
  Arm1/1 -> [Arm], Bus Selector1/1
  Bus Selector1/1 -> [ArmL]  "<cg2motor_arm4_m>"
  [ArmL] -> 3x3 Cross Product1/1
  Environment/1 -> Bus Selector2/1
  Bus Selector2/1 -> [rho]  "<air_density_kgm3>"
  [rho] -> Forces/4(rho)
  [Arm] -> Subsystem/4(Arm)
  [Arm] -> Forces/5(Arm)
  [rho] -> Moments/1(rho)
  [Arm] -> Moments/3(Arm)
  Motor_RPM/1 -> Gain/1
  Gain/1 -> [w_rads]
  [w_rads] -> Subsystem/3(w)
  [w_rads] -> Moments/2(w)
  [w_rads] -> Forces/3(w)
  Bus Selector/1 -> [Vb_ms]  "<vel_b_ms>"
  Bus Selector/2 -> [pqr_rads]  "<angular_vel_b_rads>"
  [pqr_rads] -> Subsystem/2(pqr)
  [Vb_ms] -> Subsystem/1(Vb)
  [Iz_prop_kgm2] -> Product2/2
  Product/1 -> Gain1/1
  [w_rads] -> Derivative/1, Product1/2, Product/1
  Product2/1 -> Gain2/1
  Product1/1 -> Mux/1
  Selector/1 -> Product/2
  Mux/1 -> Product2/1
  [pqr_rads] -> Selector1/1, Selector/1
  Gain1/1 -> Mux/2
  Selector1/1 -> Product1/1
  Derivative/1 -> Transfer Fcn/1
  3x3 Cross Product1/1 -> Sum4/2  "tau"
  Moments/1(Mxyz) -> Sum4/3
  Bus Selector1/2 -> [Iz_prop_kgm2]  "<prop4_Izz_kgm2>"
  Transfer Fcn/1 -> Mux/3
  Gain2/1 -> Sum4/1

== system Quad_F450_Model/DYNAMIC_MODEL/Motor Forces and Moments/Motor 1/Forces ==
  note: $-sin(a_{1s})cos(b_{1s}) \\ sin(b_{1s}) \\ -cos(a_{1s})cos(b_{1s})$
  a1s : Inport
  b1s : Inport  Port=2
  w : Inport  Port=3
  rho : Inport  Port=4
  Arm : Inport  Port=5
  Bus Selector : BusSelector  OutputSignals=prop1_ct,prop1_radius_m,arm1_defect_rad
  Constant : Constant  Value=pi
  Cos : Trigonometry  Operator=cos
  Gain1 : Gain  Gain=-1
  Gain2 : Gain  Gain=-1
  Math Function3 : Math  Operator=square  SignedPower=on
  Matrix Multiply : Product  Multiplication=Matrix(*)
  Mux : Mux  Inputs=3
  Product{,2..4,6} (5 alike) : Product
  Product1 : Product  Inputs=4
  Rotation Angles to Direction Cosine Matrix : sharedtransform/Rotation Angles to Direction Cosine Matrix  rotationOrder=ZYX  aMode=aMode
  Scope : Scope  NumInputPorts=2
  Selector : Selector  InputPortWidth=3  IndexOptions=Index vector (dialog)  Indices=[3 2 1]  OutputSizes=1
  Square : Math  Operator=square
  Transpose : Math  Operator=transpose
  Trigonometric Function3 : Trigonometry  Operator=sincos
  Trigonometric Function4 : Trigonometry  Operator=sincos
  Fxyz : Outport
  wires:
  w/1 -> Math Function3/1
  Trigonometric Function3/1 -> Product2/1
  Cos/1 -> Gain1/1
  Mux/1 -> Product4/1
  Trigonometric Function4/2 -> Product3/1
  Trigonometric Function3/2 -> Gain2/1
  Product3/1 -> Mux/3
  a1s/1 -> Trigonometric Function3/1
  Trigonometric Function4/1 -> Mux/2
  Product2/1 -> Mux/1
  Gain1/1 -> Product2/2
  b1s/1 -> Cos/1, Trigonometric Function4/1
  Gain2/1 -> Product3/2
  rho/1 -> Product6/1
  Math Function3/1 -> Product/1
  Product/1 -> Product6/2
  Square/1 -> Product1/4, Product1/3
  [R] -> Square/1
  [CT] -> Product1/1
  Constant/1 -> Product1/2
  Product1/1 -> [b_rads]
  [b_rads] -> Product/2
  Arm/1 -> Bus Selector/1
  Bus Selector/1 -> [CT]  "<prop1_ct>"
  Bus Selector/2 -> [R]  "<prop1_radius_m>"
  Rotation Angles to Direction Cosine Matrix/1 -> Transpose/1
  Bus Selector/3 -> [def_rad]  "<arm1_defect_rad>"
  [def_rad] -> Selector/1
  Transpose/1 -> Matrix Multiply/1
  Selector/1 -> Rotation Angles to Direction Cosine Matrix/1
  Matrix Multiply/1 -> Scope/1, Fxyz/1
  Product6/1 -> Product4/2
  Product4/1 -> Scope/2, Matrix Multiply/2

== system Quad_F450_Model/DYNAMIC_MODEL/Motor Forces and Moments/Motor 1/Moments ==
  rho : Inport
  w : Inport  Port=2
  Arm : Inport  Port=3
  Abs1 : Abs  SaturateOnIntegerOverflow=off
  Bus Selector : BusSelector  OutputSignals=prop1_cq,prop1_radius_m
  Constant : Constant  Value=pi
  Gain : Gain  Gain=-1
  Mxy : Constant  Value=[0 0]
  Product : Product  Inputs=5
  Product1 : Product
  Product5 : Product
  Product7 : Product
  Scope : Scope
  Square : Math  Operator=square
  Vector Concatenate3 : Concatenate
  Mxyz : Outport
  wires:
  Product1/1 -> Product7/2
  Mxy/1 -> Vector Concatenate3/1
  rho/1 -> Product7/1
  Product7/1 -> Vector Concatenate3/2
  Abs1/1 -> Product5/2
  w/1 -> Abs1/1, Product5/1
  Vector Concatenate3/1 -> Mxyz/1
  [CQ] -> Product/1
  Constant/1 -> Product/2
  [R] -> Product/5, Square/1
  Square/1 -> Product/3, Product/4
  Product/1 -> Gain/1
  Product5/1 -> Product1/1
  Gain/1 -> [d_rads]
  [d_rads] -> Scope/1, Product1/2
  Arm/1 -> Bus Selector/1
  Bus Selector/1 -> [CQ]  "<prop1_cq>"
  Bus Selector/2 -> [R]  "<prop1_radius_m>"

== system Quad_F450_Model/DYNAMIC_MODEL/Motor Forces and Moments/Motor 1/Subsystem ==
  Vb : Inport
  pqr : Inport  Port=2
  w : Inport  Port=3
  Arm : Inport  Port=4
  3x3 Cross Product : sharedutil/3x3 Cross Product  aMode=aMode
  Add : Sum
  Bus Selector : BusSelector  OutputSignals=cg2motor_arm1_m
  Demux : Demux  Outputs=2
  Gain : Gain  Gain=Copter.blade_flap_active
  J : Subsystem
  Sum : aerolibpropulsionsys/Flap/Sum  Inputs=++|  CollapseDim=1  OutMin=[]  OutMax=[]  SampleTime=-1
  beta1 : Subsystem
  beta2 : Subsystem
  lc and mu : Subsystem
  a1s : Outport
  b1s : Outport  Port=2
  wires:
  w/1 -> beta2/2(w), beta1/4(w), lc and mu/2(w)
  Sum/1 -> lc and mu/1(Vr), J/1(Vr)  "Vr"
  Demux/1 -> a1s/1
  beta1/1(beta1) -> Add/1
  Add/1 -> Gain/1  "beta"
  pqr/1 -> beta2/3(pqr), 3x3 Cross Product/1
  beta2/1(beta2) -> Add/2
  Arm/1 -> Bus Selector/1, beta1/5(Arm), beta2/4(Arm), lc and mu/3(Arm)
  lc and mu/2(mu) -> beta2/1(mu), beta1/3(mu)
  lc and mu/1(lc) -> beta1/2(lc)
  Demux/2 -> b1s/1
  3x3 Cross Product/1 -> Sum/2
  Vb/1 -> Sum/1
  Bus Selector/1 -> 3x3 Cross Product/2  "<cg2motor_arm1_m>"
  J/1(J) -> beta1/1(J)
  Gain/1 -> Demux/1

== system Quad_F450_Model/DYNAMIC_MODEL/Motor Forces and Moments/Motor 2/Forces ==
  a1s : Inport
  b1s : Inport  Port=2
  w : Inport  Port=3
  rho : Inport  Port=4
  Arm : Inport  Port=5
  Bus Selector : BusSelector  OutputSignals=prop2_ct,prop2_radius_m,arm2_defect_rad
  Constant : Constant  Value=pi
  Cos : Trigonometry  Operator=cos
  Gain1 : Gain  Gain=-1
  Gain2 : Gain  Gain=-1
  Math Function3 : Math  Operator=square  SignedPower=on
  Matrix Multiply : Product  Multiplication=Matrix(*)
  Mux : Mux  Inputs=3
  Product{,2..4,6} (5 alike) : Product
  Product1 : Product  Inputs=4
  Rotation Angles to Direction Cosine Matrix : sharedtransform/Rotation Angles to Direction Cosine Matrix  rotationOrder=ZYX  aMode=aMode
  Selector : Selector  InputPortWidth=3  IndexOptions=Index vector (dialog)  Indices=[3 2 1]  OutputSizes=1
  Square : Math  Operator=square
  Transpose : Math  Operator=transpose
  Trigonometric Function3 : Trigonometry  Operator=sincos
  Trigonometric Function4 : Trigonometry  Operator=sincos
  Fxyz : Outport
  wires:
  w/1 -> Math Function3/1
  Trigonometric Function3/1 -> Product2/1
  Cos/1 -> Gain1/1
  Mux/1 -> Product4/1
  Trigonometric Function4/2 -> Product3/1
  Trigonometric Function3/2 -> Gain2/1
  Product3/1 -> Mux/3
  a1s/1 -> Trigonometric Function3/1
  Trigonometric Function4/1 -> Mux/2
  Product2/1 -> Mux/1
  Gain1/1 -> Product2/2
  b1s/1 -> Cos/1, Trigonometric Function4/1
  Product6/1 -> Product4/2
  Gain2/1 -> Product3/2
  rho/1 -> Product6/1
  Math Function3/1 -> Product/1
  Product/1 -> Product6/2
  Square/1 -> Product1/4, Product1/3
  [R] -> Square/1
  [CT] -> Product1/1
  Constant/1 -> Product1/2
  Product1/1 -> [b_rads]
  [b_rads] -> Product/2
  Arm/1 -> Bus Selector/1
  Bus Selector/1 -> [CT]  "<prop2_ct>"
  Bus Selector/2 -> [R]  "<prop2_radius_m>"
  Transpose/1 -> Matrix Multiply/1
  Matrix Multiply/1 -> Fxyz/1
  Selector/1 -> Rotation Angles to Direction Cosine Matrix/1
  [def_rad] -> Selector/1
  Rotation Angles to Direction Cosine Matrix/1 -> Transpose/1
  Product4/1 -> Matrix Multiply/2
  Bus Selector/3 -> [def_rad]  "<arm2_defect_rad>"

== system Quad_F450_Model/DYNAMIC_MODEL/Motor Forces and Moments/Motor 2/Moments ==
  rho : Inport
  w : Inport  Port=2
  Arm : Inport  Port=3
  Abs1 : Abs  SaturateOnIntegerOverflow=off
  Bus Selector : BusSelector  OutputSignals=prop2_cq,prop2_radius_m
  Constant : Constant  Value=pi
  Gain : Gain  Gain=-1
  Mxy : Constant  Value=[0 0]
  Product : Product  Inputs=5
  Product1 : Product
  Product5 : Product
  Product7 : Product
  Square : Math  Operator=square
  Vector Concatenate3 : Concatenate
  Mxyz : Outport
  wires:
  Product1/1 -> Product7/2
  Mxy/1 -> Vector Concatenate3/1
  rho/1 -> Product7/1
  Product7/1 -> Vector Concatenate3/2
  Abs1/1 -> Product5/2
  w/1 -> Abs1/1, Product5/1
  Vector Concatenate3/1 -> Mxyz/1
  [CQ] -> Product/1
  Constant/1 -> Product/2
  [R] -> Product/5, Square/1
  Square/1 -> Product/3, Product/4
  Product/1 -> Gain/1
  Product5/1 -> Product1/1
  Gain/1 -> [d_rads]
  [d_rads] -> Product1/2
  Arm/1 -> Bus Selector/1
  Bus Selector/1 -> [CQ]  "<prop2_cq>"
  Bus Selector/2 -> [R]  "<prop2_radius_m>"

== system Quad_F450_Model/DYNAMIC_MODEL/Motor Forces and Moments/Motor 2/Subsystem ==
  Vb : Inport
  pqr : Inport  Port=2
  w : Inport  Port=3
  Arm : Inport  Port=4
  3x3 Cross Product : sharedutil/3x3 Cross Product  aMode=aMode
  Add : Sum
  Bus Selector : BusSelector  OutputSignals=cg2motor_arm2_m
  Demux : Demux  Outputs=2
  Gain : Gain  Gain=Copter.blade_flap_active
  J : Subsystem
  Sum : aerolibpropulsionsys/Flap/Sum  Inputs=++|  CollapseDim=1  OutMin=[]  OutMax=[]  SampleTime=-1
  beta1 : Subsystem
  beta2 : Subsystem
  lc and mu : Subsystem
  a1s : Outport
  b1s : Outport  Port=2
  wires:
  w/1 -> beta2/2(w), beta1/4(w), lc and mu/2(w)
  Sum/1 -> lc and mu/1(Vr), J/1(Vr)  "Vr"
  Demux/1 -> a1s/1
  beta1/1(beta1) -> Add/1
  Add/1 -> Gain/1  "beta"
  pqr/1 -> beta2/3(pqr), 3x3 Cross Product/1
  beta2/1(beta2) -> Add/2
  Arm/1 -> Bus Selector/1, beta1/5(Arm), beta2/4(Arm), lc and mu/3(Arm)
  lc and mu/2(mu) -> beta2/1(mu), beta1/3(mu)
  lc and mu/1(lc) -> beta1/2(lc)
  Demux/2 -> b1s/1
  3x3 Cross Product/1 -> Sum/2
  Vb/1 -> Sum/1
  Bus Selector/1 -> 3x3 Cross Product/2  "<cg2motor_arm2_m>"
  J/1(J) -> beta1/1(J)
  Gain/1 -> Demux/1

== system Quad_F450_Model/DYNAMIC_MODEL/Motor Forces and Moments/Motor 3/Forces ==
  a1s : Inport
  b1s : Inport  Port=2
  w : Inport  Port=3
  rho : Inport  Port=4
  Arm : Inport  Port=5
  Bus Selector : BusSelector  OutputSignals=prop3_ct,prop3_radius_m,arm3_defect_rad
  Constant : Constant  Value=pi
  Cos : Trigonometry  Operator=cos
  Gain1 : Gain  Gain=-1
  Gain2 : Gain  Gain=-1
  Math Function3 : Math  Operator=square  SignedPower=on
  Matrix Multiply : Product  Multiplication=Matrix(*)
  Mux : Mux  Inputs=3
  Product{,2..4,6} (5 alike) : Product
  Product1 : Product  Inputs=4
  Rotation Angles to Direction Cosine Matrix : sharedtransform/Rotation Angles to Direction Cosine Matrix  rotationOrder=ZYX  aMode=aMode
  Selector : Selector  InputPortWidth=3  IndexOptions=Index vector (dialog)  Indices=[3 2 1]  OutputSizes=1
  Square : Math  Operator=square
  Transpose : Math  Operator=transpose
  Trigonometric Function3 : Trigonometry  Operator=sincos
  Trigonometric Function4 : Trigonometry  Operator=sincos
  Fxyz : Outport
  wires:
  w/1 -> Math Function3/1
  Trigonometric Function3/1 -> Product2/1
  Cos/1 -> Gain1/1
  Mux/1 -> Product4/1
  Trigonometric Function4/2 -> Product3/1
  Trigonometric Function3/2 -> Gain2/1
  Product3/1 -> Mux/3
  a1s/1 -> Trigonometric Function3/1
  Trigonometric Function4/1 -> Mux/2
  Product2/1 -> Mux/1
  Gain1/1 -> Product2/2
  b1s/1 -> Cos/1, Trigonometric Function4/1
  Product6/1 -> Product4/2
  Gain2/1 -> Product3/2
  rho/1 -> Product6/1
  Math Function3/1 -> Product/1
  Product/1 -> Product6/2
  Square/1 -> Product1/4, Product1/3
  [R] -> Square/1
  [CT] -> Product1/1
  Constant/1 -> Product1/2
  Product1/1 -> [b_rads]
  [b_rads] -> Product/2
  Arm/1 -> Bus Selector/1
  Bus Selector/1 -> [CT]  "<prop3_ct>"
  Bus Selector/2 -> [R]  "<prop3_radius_m>"
  Transpose/1 -> Matrix Multiply/1
  Matrix Multiply/1 -> Fxyz/1
  Selector/1 -> Rotation Angles to Direction Cosine Matrix/1
  [def_rad] -> Selector/1
  Rotation Angles to Direction Cosine Matrix/1 -> Transpose/1
  Product4/1 -> Matrix Multiply/2
  Bus Selector/3 -> [def_rad]  "<arm3_defect_rad>"

== system Quad_F450_Model/DYNAMIC_MODEL/Motor Forces and Moments/Motor 3/Moments ==
  rho : Inport
  w : Inport  Port=2
  Arm : Inport  Port=3
  Abs1 : Abs  SaturateOnIntegerOverflow=off
  Bus Selector : BusSelector  OutputSignals=prop3_cq,prop3_radius_m
  Constant : Constant  Value=pi
  Gain : Gain  Gain=-1
  Mxy : Constant  Value=[0 0]
  Product : Product  Inputs=5
  Product1 : Product
  Product5 : Product
  Product7 : Product
  Square : Math  Operator=square
  Vector Concatenate3 : Concatenate
  Mxyz : Outport
  wires:
  Product1/1 -> Product7/2
  Mxy/1 -> Vector Concatenate3/1
  rho/1 -> Product7/1
  Product7/1 -> Vector Concatenate3/2
  Abs1/1 -> Product5/2
  w/1 -> Abs1/1, Product5/1
  Vector Concatenate3/1 -> Mxyz/1
  [CQ] -> Product/1
  Constant/1 -> Product/2
  [R] -> Product/5, Square/1
  Square/1 -> Product/3, Product/4
  Product/1 -> Gain/1
  Product5/1 -> Product1/1
  Gain/1 -> [d_rads]
  [d_rads] -> Product1/2
  Arm/1 -> Bus Selector/1
  Bus Selector/1 -> [CQ]  "<prop3_cq>"
  Bus Selector/2 -> [R]  "<prop3_radius_m>"

== system Quad_F450_Model/DYNAMIC_MODEL/Motor Forces and Moments/Motor 3/Subsystem ==
  Vb : Inport
  pqr : Inport  Port=2
  w : Inport  Port=3
  Arm : Inport  Port=4
  3x3 Cross Product : sharedutil/3x3 Cross Product  aMode=aMode
  Add : Sum
  Bus Selector : BusSelector  OutputSignals=cg2motor_arm3_m
  Demux : Demux  Outputs=2
  Gain : Gain  Gain=Copter.blade_flap_active
  J : Subsystem
  Sum : aerolibpropulsionsys/Flap/Sum  Inputs=++|  CollapseDim=1  OutMin=[]  OutMax=[]  SampleTime=-1
  beta1 : Subsystem
  beta2 : Subsystem
  lc and mu : Subsystem
  a1s : Outport
  b1s : Outport  Port=2
  wires:
  w/1 -> beta2/2(w), beta1/4(w), lc and mu/2(w)
  Sum/1 -> lc and mu/1(Vr), J/1(Vr)  "Vr"
  Demux/1 -> a1s/1
  beta1/1(beta1) -> Add/1
  Add/1 -> Gain/1  "beta"
  pqr/1 -> beta2/3(pqr), 3x3 Cross Product/1
  beta2/1(beta2) -> Add/2
  Arm/1 -> Bus Selector/1, beta1/5(Arm), beta2/4(Arm), lc and mu/3(Arm)
  lc and mu/2(mu) -> beta2/1(mu), beta1/3(mu)
  lc and mu/1(lc) -> beta1/2(lc)
  Demux/2 -> b1s/1
  3x3 Cross Product/1 -> Sum/2
  Vb/1 -> Sum/1
  Bus Selector/1 -> 3x3 Cross Product/2  "<cg2motor_arm3_m>"
  J/1(J) -> beta1/1(J)
  Gain/1 -> Demux/1

== system Quad_F450_Model/DYNAMIC_MODEL/Motor Forces and Moments/Motor 4/Forces ==
  a1s : Inport
  b1s : Inport  Port=2
  w : Inport  Port=3
  rho : Inport  Port=4
  Arm : Inport  Port=5
  Bus Selector : BusSelector  OutputSignals=prop4_ct,prop4_radius_m,arm4_defect_rad
  Constant : Constant  Value=pi
  Cos : Trigonometry  Operator=cos
  Gain1 : Gain  Gain=-1
  Gain2 : Gain  Gain=-1
  Math Function3 : Math  Operator=square  SignedPower=on
  Matrix Multiply : Product  Multiplication=Matrix(*)
  Mux : Mux  Inputs=3
  Product{,2..4,6} (5 alike) : Product
  Product1 : Product  Inputs=4
  Rotation Angles to Direction Cosine Matrix : sharedtransform/Rotation Angles to Direction Cosine Matrix  rotationOrder=ZYX  aMode=aMode
  Selector : Selector  InputPortWidth=3  IndexOptions=Index vector (dialog)  Indices=[3 2 1]  OutputSizes=1
  Square : Math  Operator=square
  Transpose : Math  Operator=transpose
  Trigonometric Function3 : Trigonometry  Operator=sincos
  Trigonometric Function4 : Trigonometry  Operator=sincos
  Fxyz : Outport
  wires:
  w/1 -> Math Function3/1
  Trigonometric Function3/1 -> Product2/1
  Cos/1 -> Gain1/1
  Mux/1 -> Product4/1
  Trigonometric Function4/2 -> Product3/1
  Trigonometric Function3/2 -> Gain2/1
  Product3/1 -> Mux/3
  a1s/1 -> Trigonometric Function3/1
  Trigonometric Function4/1 -> Mux/2
  Product2/1 -> Mux/1
  Gain1/1 -> Product2/2
  b1s/1 -> Cos/1, Trigonometric Function4/1
  Product6/1 -> Product4/2
  Gain2/1 -> Product3/2
  rho/1 -> Product6/1
  Math Function3/1 -> Product/1
  Product/1 -> Product6/2
  Square/1 -> Product1/4, Product1/3
  [R] -> Square/1
  [CT] -> Product1/1
  Constant/1 -> Product1/2
  Product1/1 -> [b_rads]
  [b_rads] -> Product/2
  Arm/1 -> Bus Selector/1
  Bus Selector/1 -> [CT]  "<prop4_ct>"
  Bus Selector/2 -> [R]  "<prop4_radius_m>"
  Transpose/1 -> Matrix Multiply/1
  Matrix Multiply/1 -> Fxyz/1
  Selector/1 -> Rotation Angles to Direction Cosine Matrix/1
  [def_rad] -> Selector/1
  Rotation Angles to Direction Cosine Matrix/1 -> Transpose/1
  Product4/1 -> Matrix Multiply/2
  Bus Selector/3 -> [def_rad]  "<arm4_defect_rad>"
